simulink model "cantharide"  (Simulink 7.9)
settings: Solver=ode45  StartTime=0.0  StopTime=2  RelTol=1e-3
model workspace (MATLAB code in the model file):
  | FlySpeed = 80;
libraries: simulink x1
settings Model: Creator=tbourke  LastModifiedBy=tbourke
settings GRTTargetCC: CombineOutputUpdateFcns=off  GRTInterface=on

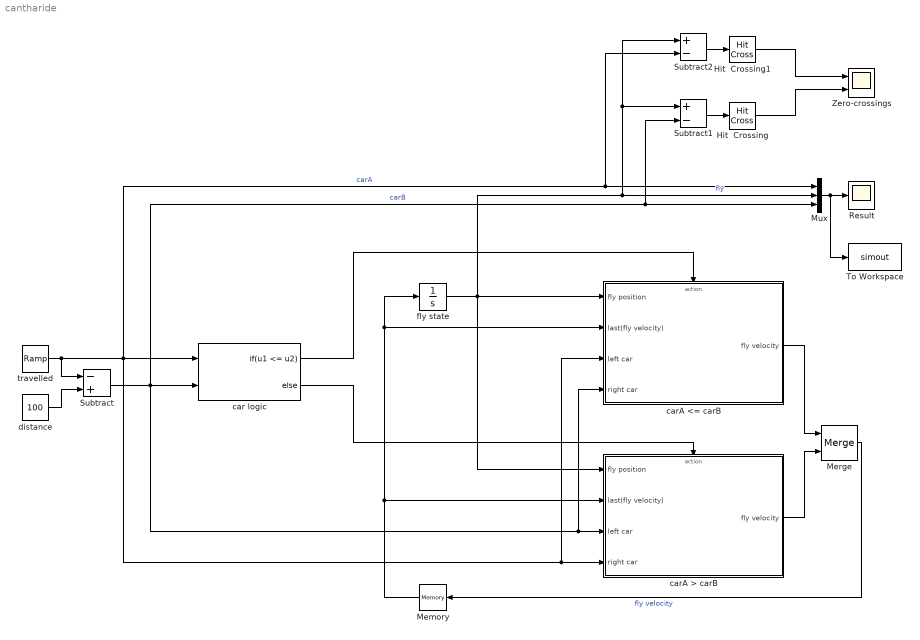
== system cantharide ==
  Hit  Crossing : HitCross
  Hit  Crossing1 : HitCross
  Memory : Memory
  Merge : Merge
  Mux : Mux  Inputs=3
  Result : Scope
      settings: TimeRange=2  YMin=0  YMax=100  MaxDataPoints=500000  SampleInput=on
  Subtract : Sum  Inputs=-+
  Subtract1 : Sum  Inputs=+-
  Subtract2 : Sum  Inputs=+-
  To Workspace : ToWorkspace  VariableName=simout  SampleTime=-1
  Zero-crossings : Scope  NumInputPorts=2
      settings: TimeRange=2  YMin=0~0  YMax=1~1  MaxDataPoints=500000  SampleInput=on
  car logic : If  NumInputs=2  IfExpression=u1 <= u2  ZeroCross=off
  carA <= carB : Subsystem  TreatAsAtomicUnit=on
  carA > carB : Subsystem  TreatAsAtomicUnit=on
  distance : Constant  Value=100
  fly state : Integrator
  travelled : simulink/Sources/Ramp  slope=50  start=0  X0=0
  wires:
  distance/1 -> Subtract/2
  travelled/1 -> Subtract/1, car logic/1, carA > carB/4(right car), carA <= carB/3(left car), Mux/1, Subtract2/2  "carA"
  Mux/1 -> Result/1, To Workspace/1
  Subtract/1 -> car logic/2, carA > carB/3(left car), carA <= carB/4(right car), Mux/3, Subtract1/2  "carB"
  car logic/1 -> carA <= carB/Action
  car logic/2 -> carA > carB/Action
  carA <= carB/1(fly velocity) -> Merge/1
  carA > carB/1(fly velocity) -> Merge/2
  Merge/1 -> Memory/1  "fly velocity"
  fly state/1 -> carA <= carB/1(fly position), carA > carB/1(fly position), Mux/2, Subtract1/1, Subtract2/1  "fly"
  Memory/1 -> carA > carB/2(last(fly velocity)), fly state/1, carA <= carB/2(last(fly velocity))
  Subtract1/1 -> Hit  Crossing/1
  Subtract2/1 -> Hit  Crossing1/1
  Hit  Crossing1/1 -> Zero-crossings/1
  Hit  Crossing/1 -> Zero-crossings/2

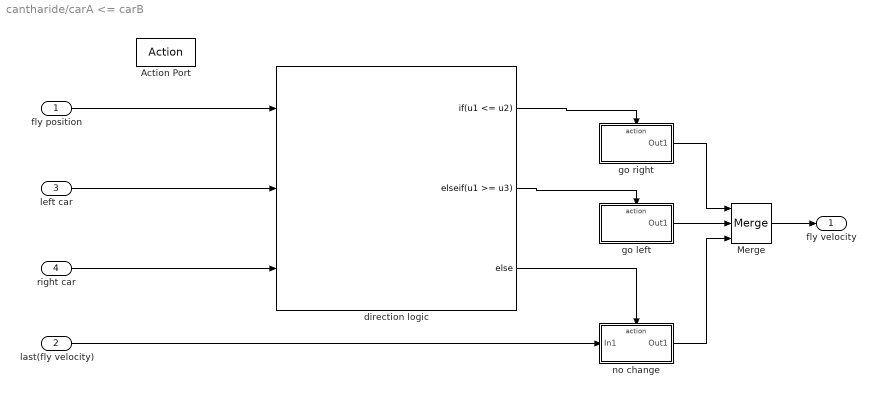
== system cantharide/carA <= carB ==
  fly position : Inport
  last(fly velocity) : Inport  Port=2
  left car : Inport  Port=3
  right car : Inport  Port=4
  Action Port : ActionPort  ActionType=then
  Merge : Merge  Inputs=3  InitialOutput=80
  direction logic : If  NumInputs=3  IfExpression=u1 <= u2  ElseIfExpressions=u1 >= u3
  go left : Subsystem  TreatAsAtomicUnit=on
  go right : Subsystem  TreatAsAtomicUnit=on
  no change : Subsystem  TreatAsAtomicUnit=on
  fly velocity : Outport
  wires:
  fly position/1 -> direction logic/1
  left car/1 -> direction logic/2
  right car/1 -> direction logic/3
  direction logic/1 -> go right/Action
  direction logic/2 -> go left/Action
  last(fly velocity)/1 -> no change/1(In1)
  direction logic/3 -> no change/Action
  Merge/1 -> fly velocity/1
  go right/1(Out1) -> Merge/1
  go left/1(Out1) -> Merge/2
  no change/1(Out1) -> Merge/3

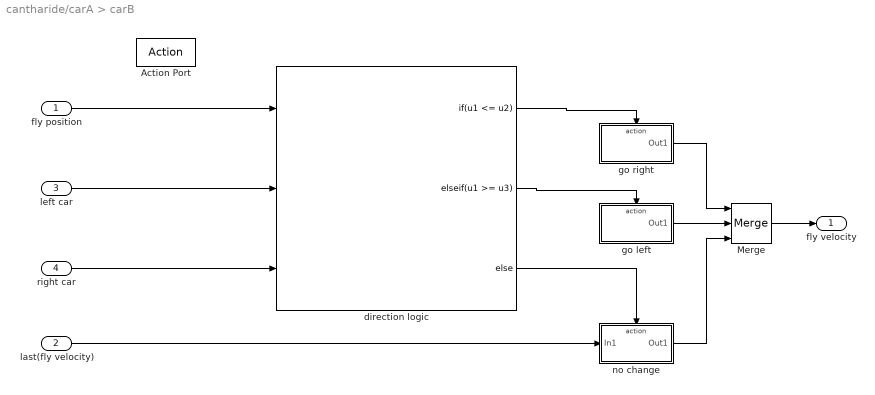
== system cantharide/carA > carB ==
  fly position : Inport
  last(fly velocity) : Inport  Port=2
  left car : Inport  Port=3
  right car : Inport  Port=4
  Action Port : ActionPort  ActionType=else
  Merge : Merge  Inputs=3  InitialOutput=80
  direction logic : If  NumInputs=3  IfExpression=u1 <= u2  ElseIfExpressions=u1 >= u3
  go left : Subsystem  TreatAsAtomicUnit=on
  go right : Subsystem  TreatAsAtomicUnit=on
  no change : Subsystem  TreatAsAtomicUnit=on
  fly velocity : Outport
  wires:
  fly position/1 -> direction logic/1
  left car/1 -> direction logic/2
  right car/1 -> direction logic/3
  direction logic/1 -> go right/Action
  direction logic/2 -> go left/Action
  last(fly velocity)/1 -> no change/1(In1)
  direction logic/3 -> no change/Action
  Merge/1 -> fly velocity/1
  go right/1(Out1) -> Merge/1
  go left/1(Out1) -> Merge/2
  no change/1(Out1) -> Merge/3

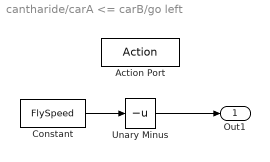
== system cantharide/carA <= carB/go left ==
  Action Port : ActionPort  ActionType=elseif
  Constant : Constant  Value=FlySpeed
  Unary Minus : UnaryMinus
  Out1 : Outport
  wires:
  Unary Minus/1 -> Out1/1
  Constant/1 -> Unary Minus/1

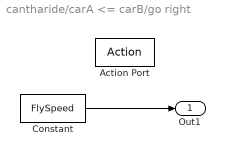
== system cantharide/carA <= carB/go right ==
  Action Port : ActionPort  ActionType=then
  Constant : Constant  Value=FlySpeed
  Out1 : Outport
  wires:
  Constant/1 -> Out1/1

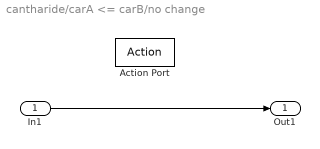
== system cantharide/carA <= carB/no change ==
  In1 : Inport
  Action Port : ActionPort  ActionType=else
  Out1 : Outport
  wires:
  In1/1 -> Out1/1

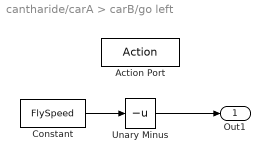
== system cantharide/carA > carB/go left ==
  Action Port : ActionPort  ActionType=elseif
  Constant : Constant  Value=FlySpeed
  Unary Minus : UnaryMinus
  Out1 : Outport
  wires:
  Unary Minus/1 -> Out1/1
  Constant/1 -> Unary Minus/1

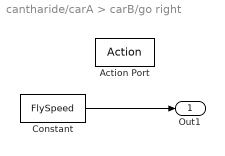
== system cantharide/carA > carB/go right ==
  Action Port : ActionPort  ActionType=then
  Constant : Constant  Value=FlySpeed
  Out1 : Outport
  wires:
  Constant/1 -> Out1/1

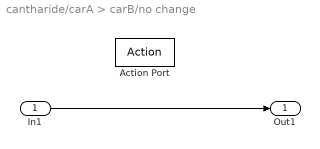
== system cantharide/carA > carB/no change ==
  In1 : Inport
  Action Port : ActionPort  ActionType=else
  Out1 : Outport
  wires:
  In1/1 -> Out1/1
